simulink model "Actuator_Bench_CAN"  (R2014b)
settings: Solver=ode4  StartTime=0.0  StopTime=Inf  FixedStep=0.001  RelTol=1e-3
PostLoadFcn:
  | , if any(exist('dsrtsu_mdlpostloadfcn', 'file') == [2, 3, 6]), try dsrtsu_mdlpostloadfcn('Execute', bdroot); catch fprintf('Error in PostLoadFcn (dsrtsu_mdlpostloadfcn) for model "%s":\n %s\n', bdroot, lasterr); end, end,
undefined symbols (not defined in the file or in its folder): rticanmm_blockfcn, rticanmm_initfcn
libraries: rtimmsu_dsrtlib x2
settings Model: DSRTSU_INTERNAL_RTI_VER=450  DSRTSU_INTERNAL_RTI_TYPE=rti1401  RTICANMMDATA=struct('GeneralSetupData',struct('modelroot','F:\Clutch','generalsettings',struct('filesettings',struct('destfolder',struct('Name','RTICANMM_FILES','Check',1),'buildfolder',struct('Name','.','Check',1),'AbsDestfolder',struct('Name','F:\Clutch\RTICANMM_FILES'),'AbsBuildfolder',struct('Name','F:\Clutch'))),'options',struct('addpaths',1,'rmpaths',1,'addtrcexclusion',logical(1),'cannavigator',struct('checkmonitoring',0,'checkinternmonitoring',1,'serviceno','31','hostservicedefheader',struct('name','RTICANMMHostService_Lesson1_TutorialModel.h','path','E:\Lessons_Tutorial\Lesson1_results\RTICANMMTutorial\RTICANMM_FILES\RTICANMMHostService_Lesson1_TutorialModel.h')),'show_usrtrc',0,'use_usrtrc',0,'addpath2usrmk',1),'advanced',struct('options',[1 1 1 1 1 1 1 1 1 1 1 1 1 1 1 1 1 1 1 1 1 1 1 1 1 1 1 1 1 1 1 1 1 1 1 1 1 1 1 1 1 1 1 1 1 1 1 1 1 1 1 1 1 1 1 1 1 1 1 1 1 1 1 1 1 1 1 1 1 1 1 1 1 1 1 1 1 1 1 1 1 1 1 1 1 1 1 1 1 1 1 1 1 1 1 1 1 1 1 1]),'MPSetup',{{}},'modelname','Actuator_Bench_CAN2','blockdata',struct('generalsettings',struct('filesettings',struct('destfolder',struct('Name','.','Check',1),'AbsDestfolder',struct('Name','T:\TOOL_SOURCES\CANnedy\m'),'buildfolder',struct('Name','.','Check',1),'AbsBuildfolder',struct('Name','C:\MATLAB6p5\work'))),'options',struct('addpaths',1,'rmpaths',1,'addpath2usrmk',1),'modelname','rticanmmlib','modelroot','T:\TOOL_SOURCES\CANnedy\m'),'userdata',struct('CANMMName',{{'Chassis_M1','Chassis_M2'}},'HostServiceChannelID',{{'ACTUATOR_CAN',[],[],[],[]}}),'RTI',struct('Type','RTI1401','Ver','7.3','Date','02-Nov-2014'),'version','4.0.735878.5444907408','MMType','RTICANMM','block',['Actuator_Bench_CAN2/RTICANMM' char(10) 'GeneralSetup']))  DSRTSU_INTERNAL_RTIFPGA=40  BufferReuse=off  Creator=Burninator  LastModifiedBy=Stealth
settings OptimizationCC: BlockReduction=off  OptimizeBlockIOStorage=off  BufferReuse=off  GlobalBufferReuse=off  ExpressionFolding=off  LocalBlockOutputs=off
settings HardwareCC: ProdIntDivRoundTo=Zero  ProdEndianess=BigEndian  ProdHWDeviceType=Generic->Custom  TargetIntDivRoundTo=Zero  TargetEndianess=BigEndian  TargetHWDeviceType=Generic->Custom
settings RTWCC: SystemTargetFile=rti1401.tlc  MakeCommand=make_rti  TemplateMakefile=rti1401.tmf  Description=dSPACE DS1401 Hardware Platform  ProcessScript=rti1401_make_rtw_hook
settings STFCustomTargetCC: ParMdlRefBuildCompliant=on  GeneratePreprocessorConditionals=Disable all  SystemTargetFile=rti1401.tlc
settings GRTTargetCC: CompOptLevelCompliant=off  ConcurrentExecutionCompliant=off  CombineOutputUpdateFcns=off  MatFileLogging=off  CPPClassGenCompliant=off  GRTInterface=on  ExtModeMexFile=noextcomm

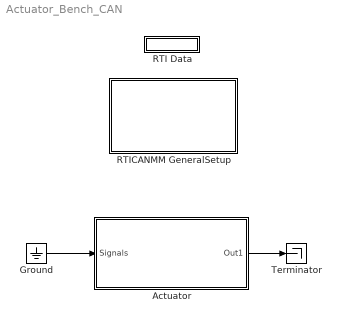
== system Actuator_Bench_CAN ==
  Actuator : Subsystem
  Ground : Ground
  RTI Data : Subsystem  Tag=struct('RTIDataServer',struct('RTIDataServerVs','2','RTIModelDescription','struct(''main'',''Actuator_Bench_CAN2'',''sub'','''',''isMp'',0)'))  LoadFcn="if exist('rtidc'), try,  rtidc('DataHostBlockClbLoad', gcbh); catch, disp(['Warning: ''LoadFcn'' for RTI Data block failed: ' lasterr]); end, end,"  mask(RTI_DATA_HOST){}
      mask help:
      | RTI Data Block.
      | This block is used by RTI to store internal model-dependent data.
      | Please keep this block on the root level of the model. Deleting this block will result in data loss.
      |
      | NEVER DELETE OR COPY THIS BLOCK!
      settings: CopyFcn="if exist('rtidc'), try,  rtidc('DataHostBlockClbCopy', gcbh); catch, disp(['Warning: ''CopyFcn'' for RTI Data block failed: ' lasterr]); end, end,"  DeleteFcn="if exist('rtidc'), try,  rtidc('DataHostBlockClbDelete', gcbh); catch, disp(['Warning: ''DeleteFcn'' for RTI Data block failed: ' lasterr]); end, end,"  ModelCloseFcn="if exist('rtidc'), try,  rtidc('DataHostBlockClbModelClose', gcbh); catch, disp(['Warning: ''ModelCloseFcn'' for RTI Data block failed: ' lasterr]); end, end,"  PreSaveFcn="if exist('rtidc'), try,  rtidc('DataHostBlockClbPreSave', gcbh); catch, disp(['Warning: ''PreSaveFcn'' for RTI Data block failed: ' lasterr]); end, end,"  PostSaveFcn="if exist('rtidc'), try,  rtidc('DataHostBlockClbPostSave', gcbh); catch, disp(['Warning: ''PostSaveFcn'' for RTI Data block failed: ' lasterr]); end, end,"  NameChangeFcn="if exist('rtidc'), try,  rtidc('DataHostBlockClbNameChange', gcbh); catch, disp(['Warning: ''NameChangeFcn'' for RTI Data block failed: ' lasterr]); end, end,"
      mask Help:
      | RTI Data Block.
      | This block is used by RTI to store internal model-dependent data.
      | Please keep this block on the root level of the model. Deleting this block will result in data loss.
      | 
      | NEVER DELETE OR COPY THIS BLOCK!
      mask Display:
      | text(0.5, 0.5, 'RTI Data', 'HorizontalAlignment', 'center');
      | plot([1 0]);
  RTICANMM GeneralSetup : Subsystem  InitFcn=rticanmm_initfcn(gcb, 'CANnedySettings')  ClipboardFcn=rticanmm_blockfcn('ClipboardFcn', 'CANnedySettings', gcb)  mask(RTICANMM){DSProperties=struct('RTI',struct('Version',uint32(1),'BlockType',struct('isSLSource',uint8(1),'isSLSink',uint8(1),'isHWSource',uint8(0),'isHWSink',uint8(0),'isSetup',uint8(0),'isInline',uint8(1),'isNonInline',uint8(0),'isInterrupt',uint8(0),'isChannelwise',uint8(0)),'IOBoardType','RTICANMM','UnitType','RTICANMM','Identifier','GENERALSETUP','DialogType','SL','BlockSet','RTICANMM','SlaveProcessor','CAN')), CANMMDestFolder=RTICANMM_FILES, CANMMBuildDir=., CANMMAddPaths=on, CANMMAddpathUserMake=on, CANMMRemovePathOnclose=on, CANMMType=CANnedySettings, CANMMProperties=struct('modelroot','F:\Clutch','generalsettings',struct('filesettings',struct('destfolder',struct('Name','RTICANMM_FILES','Check',1),'buildfolder',struct('Name','.','Check',1),'AbsDestfolder',struct('Name','F:\Clutch\RTICANMM_FILES'),'AbsBuildfolder',struct('Name','F:\Clutch'))),'options',struct('addpaths',1,'rmpaths',1,'addtrcexclusion',logical(1),'cannavigator',struct('checkmonitoring',0,'checkinternmonitoring',1,'serviceno','31','hostservicedefheader',struct('name','RTICANMMHostService_Lesson1_TutorialModel.h','path','E:\Lessons_Tutorial\Lesson1_results\RTICANMMTutorial\RTICANMM_FILES\RTICANMMHostService_Lesson1_TutorialModel.h')),'show_usrtrc',0,'use_usrtrc',0,'addpath2usrmk',1),'advanced',struct('options',[1 1 1 1 1 1 1 1 1 1 1 1 1 1 1 1 1 1 1 1 1 1 1 1 1 1 1 1 1 1 1 1 1 1 1 1 1 1 1 1 1 1 1 1 1 1 1 1 1 1 1 1 1 1 1 1 1 1 1 1 1 1 1 1 1 1 1 1 1 1 1 1 1 1 1 1 1 1 1 1 1 1 1 1 1 1 1 1 1 1 1 1 1 1 1 1 1 1 1 1]),'MPSetup',{{}},'modelname','Actuator_Bench_CAN2','blockdata',struct('generalsettings',struct('filesettings',struct('destfolder',struct('Name','.','Check',1),'AbsDestfolder',struct('Name','T:\TOOL_SOURCES\CANnedy\m'),'buildfolder',struct('Name','.','Check',1),'AbsBuildfolder',struct('Name','C:\MATLAB6p5\work'))),'options',struct('addpaths',1,'rmpaths',1,'addpath2usrmk',1),'modelname','rticanmmlib','modelroot','T:\TOOL_SOURCES\CANnedy\m'),'userdata',struct('CANMMName',{{'Chassis_M1','Chassis_M2'}},'HostServiceChannelID',{{'ACTUATOR_CAN',[],[],[],[]}}),'RTI',struct('Type','RTI1401','Ver','7.3','Date','02-Nov-2014'),'version','4.0.735878.5444907408','MMType','RTICANMM','block',['Actuator_Bench_CAN2/RTICANMM' char(10) 'GeneralSetup'])}
      mask prompts: CANMMDestFolder "Destination Folder for generated Files:"; CANMMBuildDir "Build Directory (*_usr.mk, *_usr.trc)"; CANMMAddPaths "Add Paths automatically"; CANMMAddpathUserMake "Add Paths to UserMake-File"; CANMMRemovePathOnclose "Remove added Path on ModelClose"
      mask init:
      | rticanmm_initfcn(gcb,'CANnedyGeneralSettings')
      settings: CopyFcn=rticanmm_blockfcn('CopyFcn', 'CANnedySettings', gcb)  DeleteFcn=rticanmm_blockfcn('DeleteFcn', 'CANnedySettings', gcb)  ModelCloseFcn=rticanmm_blockfcn('CloseFcn', 'CANnedyGeneralSettings', gcb)  NameChangeFcn=rticanmm_blockfcn('NameChangeFcn', 'CANnedySettings', gcb)  OpenFcn=try, rticanmm_gs_gui('create',gcb), ; catch,errordlg({lasterr, '','Please check your RTI installation.'},['Error: ' upper(bdroot)], 'replace'); end  MoveFcn=rticanmm_blockfcn('MoveFcn', 'CANnedySettings', gcb)
      mask Help: eval('rticanmm_quickstart(''create'', gcb);', 'disp(lasterr);')
      mask Display: disp(sprintf(['RTI CAN\nMultiMessage\nGeneralSetup']))
  Terminator : Terminator
  wires:
  Actuator/1(Out1) -> Terminator/1
  Ground/1 -> Actuator/1(Signals)

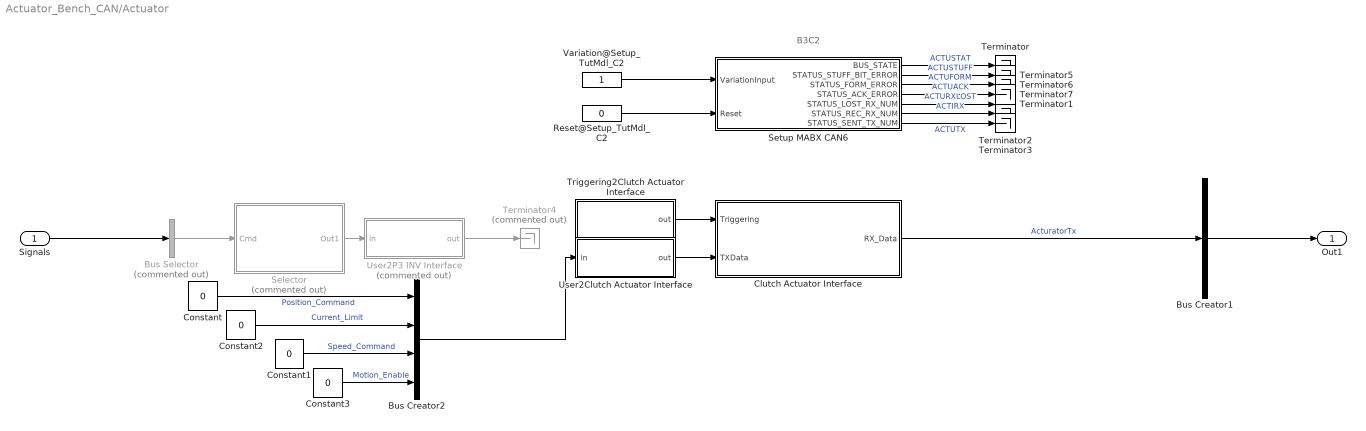
== system Actuator_Bench_CAN/Actuator ==
  note: B3C2
  Signals : Inport
  Bus Creator1 : BusCreator  Inputs=1
  Bus Creator2 : BusCreator
  Bus Selector : BusSelector  Commented=on  OutputSignals=ExecutiveCommands.ComponentStateControl.P3InvCtrl.InverterEnable[Flag],ExecutiveCommands.ComponentStateControl.P3InvCtrl.DischargeEnable[Flag],ExecutiveCommands.ComponentStateControl.P3InvCtrl.Direction[Flag],ExecutiveCommands.TorqueControl.P3Trq.P3TorqueCommand[Nm]  OutputAsBus=on
  Clutch Actuator Interface : Subsystem  InitFcn=rticanmm_blockfcn('InitFcn', 'CANnedy', gcb)  ClipboardFcn=rticanmm_blockfcn('ClipboardFcn', 'CANnedy', gcb)  mask(RTICANMM){DSProperties=struct('RTI',struct('Version',uint32(1),'BlockType',struct('isSLSource',uint8(1),'isSLSink',uint8(1),'isHWSource',uint8(0),'isHWSink',uint8(0),'isSetup',uint8(0),'isInline',uint8(1),'isNonInline',uint8(0),'isInterrupt',uint8(0),'isChannelwise',uint8(0)),'IOBoardType','RTICANMM','UnitType','RTICANMM','Identifier','Mainblock','DialogType','SL','BlockSet','RTICANMM','SlaveProcessor','CAN')), CANMMProperties=struct('RTICANMMVersion','4.0','RTICANMMVersionIntern','4.0.735878.5444907408','RTICANMMDate','02-Nov-2014','Settings','RTICANMM_MAIN_CAN6','UserTracePath','','ModelPath','F:\Clutch','filesettings',struct('FileName','Clutch.dbc','IsRelative',1,'ClusterId',1,'ClusterList',{{'default'}},'destfolder',struct('Name','RTICANMM_FILES','Check',1),'buildfolder',struct('Name','.','Check',1),'onlyfreerawcapture',0,'overlapping2variant',0,'canfdsupport',0),'onlyfreerawcapture',0,'Board',['CAN Type 1'],'BoardNum','3','ChannelNum','2','Variation','1','SetupId','ACTUATOR_CAN','MARK',['4B451E4CC965ABA1126FF18852ACAC';'52181FAC453988346E72CD977C4BB0';'1EB0637A588B713B34B1F65E3CCCD4';'7A7D1E3C4C054BB56A755C5D40C18B';'1806BA38BE006B3F777393E4A2C54E'],'date','06-Jan-2017','clock',['06.01.2017 16:38:25'],'recreate',0,'RTIVER','RTI1401','j1939',0,'TRC',struct('include',1),'rtsupport',struct('XMLFile','F:\Clutch\RTICANMM_FILES\RTICANMM_MAIN_CAN6.xml','DBCXML',struct('Path','F:\Clutch\RTICANMM_FILES\RTICANMM_MAIN_CAN6_dbc.xml','support',1,'Name','Clutch.dbc','Date',['06-Jan-2017 16:32:48'],'Type','extended','DBCSupport','ON'))), CANMMType=CANnedy, CANMMUserTraceMerged=off, CANMMUserTracePath=, CANMMChannelNum=2, CANMMBoardNum=3, CANMMDestFolder=RTICANMM_FILES, CANMMFolder=., CANMMSetupId=ACTUATOR_CAN, CANMMsave2mat=['4B451E4CC965ABA1126FF18852ACAC';'52181FAC453988346E72CD977C4BB0';'1EB0637A588B713B34B1F65E3CCCD4';'7A7D1E3C4C054BB56A755C5D40C18B';'1806BA38BE006B3F777393E4A2C54E'], CANMMName=CAN6, CANMMSettings=RTICANMM_MAIN_CAN6, CANMMIntermediateTag=RTICANMM_MAIN_CAN6_intermediate, CANMMsfcnname=RTICANMM_MAIN_CAN6}
      mask init:
      | rticanmm_initfcn(gcb, CANMMType, CANMMsfcnname)
      settings: AttributesFormatString=ACTUATOR_CAN[CAN6]: DS1401_B3_C2_V1  CopyFcn=rticanmm_blockfcn('CopyFcn', 'CANnedy', gcb)  DeleteFcn=rticanmm_blockfcn('DeleteFcn', 'CANnedy', gcb)  ModelCloseFcn=rticanmm_blockfcn('ModelCloseFcn', 'CANnedy', gcb)  NameChangeFcn=rticanmm_blockfcn('NameChangeFcn', 'CANnedy', gcb)  OpenFcn=try, rticanmm_main_gui('create',gcb); ; catch,errordlg({lasterr, '','Please check your RTI installation.'},['Error: ' upper(bdroot)], 'replace'); end  MoveFcn=rticanmm_blockfcn('MoveFcn', 'CANnedy', gcb)
      mask Help: eval('rticanmm_quickstart(''create'', gcb);', 'disp(lasterr);')
      mask Display:
      | disp(sprintf('RTI CAN\nMultiMessage\nMainSetup'))
      | port_label('input', 1, 'Triggering')
      | port_label('input', 2, 'TX Data')
      | port_label('output', 1, 'RX Data')
  Constant{,1..3} (4 alike) : Constant  Value=0
  Reset@Setup_TutMdl_C2 : Constant  Value=0  OutDataTypeStr=boolean
  Selector : Subsystem  Commented=on
  Setup MABX CAN6 : Subsystem  InitFcn=rticanmm_blockfcn('InitFcn', 'CANnedySetup', gcb)  ClipboardFcn=rticanmm_blockfcn('ClipboardFcn', 'CANnedySetup', gcb)  mask(RTICANMM){DSProperties=struct('RTI',struct('Version',uint32(1),'BlockType',struct('isSLSource',uint8(1),'isSLSink',uint8(1),'isHWSource',uint8(0),'isHWSink',uint8(0),'isSetup',uint8(0),'isInline',uint8(1),'isNonInline',uint8(0),'isInterrupt',uint8(0),'isChannelwise',uint8(0)),'IOBoardType','RTICANMM','UnitType','RTICANMM','Identifier','BUSSETUP','DialogType','SL','BlockSet','RTICANMM','SlaveProcessor','CAN')), CANMMProperties=struct('cannedy',struct('data',struct('options',struct('controllername','ACTUATOR_CAN','controllernameautomatic',[],'loglevel','0','checkrealtime',0,'checkchangebaudrate',0,'sampletime','1.000','CANControllerStatus',1,'NumberofStuffErr',1,'NumberofFormErr',1,'NumberofAckErr',1,'NumberofBit0Err',0,'NumberofsuccrecRX',1,'Numberofsuccsent',1,'NumberofBit1Err',0,'NumberofCRCErr',0,'NumberoflostRX',1,'Busoff',0,'Busload',0,'OperationPending',0,'TxRetryCount',3,'addtrcexclusion',logical(1),'cannavigator',struct('checkmonitoring',0,'checkinternmonitoring',0),'show_usrtrc',0,'use_usrtrc',0,'checkchangebaudrateFD',0),'modelroot','E:\Lessons_Tutorial\Lesson10_results\RTICANMMTutorial','generalsettings',struct('setupdata',struct('board',['CAN Type 1'],'boardno',3,'channelno',2,'Type','EXT','transceiver','ISO11898-2','busconfig','0x0','feedthrough','false','resistance',struct('r120',1,'roff',0,'r16',1,'r10',0),'baudrate','250','Frequency',[24 36],'samplemode',1,'commChannelTJA1041',6,'config',struct('standard',1,'advanced',0,'register',struct('btr0','0xC1','btr1','0x6F','sp','70','sjw','3','tseg1','15','tseg2','6','brp','1','smpl','0','btr0_36','0xC2','btr1_36','0x6F','sp_36','70','sjw_36','3','tseg1_36','15','tseg2_36','6','brp_36','2','smpl_36','0','btr0_64','0x47','btr1_64','0x1C','sp_64','87','sjw_64','1','tseg1_64','12','tseg2_64','1','brp_64','7','smpl_64','0')),'channelcfg',struct('INTENDISABLE','CAN_INT_DISABLE','intenable',0),'SETUPID','RTICANMM_ACTUATOR_CAN_ID','CONTROLLER_ID','CANMM_CTL_SETUP_ACTUATOR_CAN','mainblock_includefile','RTICANMM_SETUP_ACTUATOR_CAN','canfdenable',0,'canfdboardselected',0,'slotno',1,'moduletype','DS4342','baudrateFD','4000','termination','TERMINATION_ON'),'filesettings',struct('destfolder',struct('Name','RTICANMM_FILES','Check',1),'buildfolder',struct('Name','.','Check',1))),'advanced',struct('options',[1 1 1 1 1 1 1 1 1 1 1 1 1 1 1 1 1 1 1 1 1 1 1 1 1 1 1 1 1 1 1 1 1 1 1 1 1 1 1 1 1 1 1 1 1 1 1 1 1 1 1 1 1 1 1 1 1 1 1 1 1 1 1 1 1 1 1 1 1 1 1 1 1 1 1 1 1 1 1 1 1 1 1 1 1 1 1 1 1 1 1 1 1 1 1 1 1 1 1 1]),'partialnetdata',struct('switchedon',0,'format','STD','idmask',['XXXXX XXXXXXXX XXXXXXXX XXXXXXXX'],'idcode','0','idfilter','0','datamaskused',0,'datalength','0','datamask','0x0000000000000000','partialnetworkenable',0)),'blk',['Actuator_Bench_CAN2/Actuator/Setup MABX CAN6'],'allgeneratedfiles',{{'F:\Clutch\RTICANMM_FILES\RTICANMM_SETUP_ACTUATOR_CAN.c','F:\Clutch\RTICANMM_FILES\RTICANMM_SETUP_ACTUATOR_CAN.h','f:\clutch\rticanmm_files\rticanmm_setup_actuator_can.mexw64'}},'ismp',logical(0),'BlockDataVersion','0.7.0','recreate',0,'CANnedyTag','ACTUATOR_CAN'),'CANnedynew',0,'CANnedySettings','ACTUATOR_CAN','GeneratedFiles',{{'F:\Clutch\RTICANMM_FILES\RTICANMM_SETUP_ACTUATOR_CAN.c','F:\Clutch\RTICANMM_FILES\RTICANMM_SETUP_ACTUATOR_CAN.h','f:\clutch\rticanmm_files\rticanmm_setup_actuator_can.mexw64'}},'SFCN','RTICANMM_SETUP_ACTUATOR_CAN.c','HostService',struct('Tags',struct('DATA','RTICANMM_MonitorData','TimeStampGlobal','RTICANMM_MonitoringTimeStamp','TimeStampGlobalEnable','RTICANMM_MonitoringTimeStampEnable','Enable','CANMMMonitor_ACTUATOR_CAN','TimeStamp','MonitoringTimeStamp_ACTUATOR_CAN'),'DATA',struct('Length',18),'Info',struct('Desc',{'ID','Service','Data1','Data2','Data3','Data4','Data5','Data6','Data7','Data8','Data9','Data10','Data11','Data12','Data13','Data14','Data15','Data16'}),'Names',struct('TimeStampGlobal','TimeStamp','TimeStampGlobalEnable','TimeStamp_Enable','Enable','Monitoring_Enable','TimeStamp','Monitoring_TimeStamp'),'ChannelID',1)), CANMMType=CANnedySetup, CANMMFolder=F:\Clutch, CANMMDestFolder=RTICANMM_FILES, CANMMSettings=ACTUATOR_CAN, CANMMSFcn=RTICANMM_SETUP_ACTUATOR_CAN, CANMMBoard=DS1401, CANMMBoardNum=3, CANMMChannel=2}
      settings: AttributesFormatString=%<CANMMSettings>: %<CANMMBoard>_B%<CANMMBoardNum>_C%<CANMMChannel>  CopyFcn=rticanmm_blockfcn('CopyFcn', 'CANnedySetup', gcb)  DeleteFcn=rticanmm_blockfcn('DeleteFcn', 'CANnedySetup', gcb)  ModelCloseFcn=rticanmm_blockfcn('ModelCloseFcn', 'CANnedySetup', gcb)  NameChangeFcn=rticanmm_blockfcn('NameChangeFcn', 'CANnedySetup', gcb)  OpenFcn=try, rticanmm_setup_gui('create',gcb); ; catch,errordlg({lasterr, '','Please check your RTI installation.'},['Error: ' upper(bdroot)], 'replace'); end  MoveFcn=rticanmm_blockfcn('MoveFcn', 'CANnedySetup', gcb)
      mask Help: eval('rticanmm_quickstart(''create'', gcb);', 'disp(lasterr);')
      mask Display:
      | disp('RTI CAN\nMultiMessage\nControllerSetup')
      | 
      | port_label('input', 1 , 'Variation')
      | port_label('input', 2 , 'Reset')
      | port_label('output', 1, 'Status')
      | port_label('output', 2, 'Stuff errors')
      | port_label('output', 3, 'Format errors')
      | port_label('output', 4, 'Ack errors')
      | port_label('output', 5, 'RX lost')
      | port_label('output', 6, 'RX ok')
      | port_label('output', 7, 'TX ok')
  Terminator{,1..3,5..7} (7 alike) : Terminator
  Terminator4 : Terminator  Commented=on
  Triggering2Clutch Actuator Interface : Subsystem
      mask Display: disp('Triggering\nto RTICANMM')
  User2Clutch Actuator Interface : Subsystem
      mask Display: disp('Mapping\nto RTICANMM')
  User2P3 INV Interface : Subsystem  Commented=on
      mask Display: disp('Mapping\nto RTICANMM')
  Variation@Setup_TutMdl_C2 : Constant  OutDataTypeStr=uint8
  Out1 : Outport
  wires:
  Bus Selector/1 -> Selector/1(Cmd)
  User2P3 INV Interface/1(out) -> Terminator4/1
  Clutch Actuator Interface/1(RX_Data) -> Bus Creator1/1  "ActuratorTx"
  Signals/1 -> Bus Selector/1
  Variation@Setup_TutMdl_C2/1 -> Setup MABX CAN6/1(VariationInput)
  Reset@Setup_TutMdl_C2/1 -> Setup MABX CAN6/2(Reset)
  Bus Creator1/1 -> Out1/1
  Selector/1(Out1) -> User2P3 INV Interface/1(in)
  Setup MABX CAN6/1(BUS_STATE) -> Terminator/1  "ACTUSTAT"
  Setup MABX CAN6/5(STATUS_LOST_RX_NUM) -> Terminator1/1  "ACTURXLOST"
  Setup MABX CAN6/6(STATUS_REC_RX_NUM) -> Terminator2/1  "ACTIRX"
  Setup MABX CAN6/7(STATUS_SENT_TX_NUM) -> Terminator3/1  "ACTUTX"
  Setup MABX CAN6/4(STATUS_ACK_ERROR) -> Terminator7/1  "ACTUACK"
  Setup MABX CAN6/3(STATUS_FORM_ERROR) -> Terminator6/1  "ACTUFORM"
  Setup MABX CAN6/2(STATUS_STUFF_BIT_ERROR) -> Terminator5/1  "ACTUSTUFF"
  Constant/1 -> Bus Creator2/1  "Position_Command"
  Bus Creator2/1 -> User2Clutch Actuator Interface/1(in)
  Constant2/1 -> Bus Creator2/2  "Current_Limit"
  Constant1/1 -> Bus Creator2/3  "Speed_Command"
  Constant3/1 -> Bus Creator2/4  "Motion_Enable"
  Triggering2Clutch Actuator Interface/1(out) -> Clutch Actuator Interface/1(Triggering)
  User2Clutch Actuator Interface/1(out) -> Clutch Actuator Interface/2(TXData)

== system Actuator_Bench_CAN/RTI Data ==
  RTI Data Store : Subsystem  Tag="struct('private',struct('version',struct('dsVer',uint32(2),'dsVerCreation',uint32(2),'RTI',struct('ver','7.3','type','RTI1401')),'access',struct('type','Model','isPerm',1,'created',['06-Jan-2017 09:05:07'],'modified',['06-Jan-2017 16:41:17'],'location','')),'public',struct('main',struct('data',[]),'sub',struct('name',{{'Actuator_Bench_CAN2'}},'data',{{struct('TH',struct('thTaskInfo',struct('taskType',{'TIMER','HWINT','TMRINT','SWINT','GLINT'},'tasksNumOf',{1,0,0,0,0},'srcIds',{{'TIMERA'},{},{},{},{}},'taskNames',{{['Timer Task 1']},{},{},{},{}})),'th_tc',struct('dataType','TASK','taskGroupId','','taskGroupList',{{}},'taskSchedulingPolicy','FCFS','taskType','TIMER','blkh',-1,'srcId','TIMERA','srcSgnName',['Timer A interrupt'],'srcCpuName','','taskName',['Timer Task 1  [0.001] s'],'taskNameDisplayExt','','smplTime',0.001,'smplTimeOffs',0,'hasFixedPriority',0,'priority',1,'hasFixedOvc',0,'ovcType',1,'ovcMax',1),'tc_th',struct('dataType','TASK','taskGroupId','','taskGroupList',{{}},'taskSchedulingPolicy','FCFS','taskType','TIMER','blkh',-1,'srcId','TIMERA','srcSgnName',['Timer A interrupt'],'srcCpuName','','taskName',['Timer Task 1  [0.001] s'],'taskNameDisplayExt','','smplTime',0.001,'smplTimeOffs',0,'hasFixedPriority',0,'priority',1,'hasFixedOvc',0,'ovcType',1,'ovcMax',1))}})))"  mask(RTI_DATA_STORE){}
      mask help:
      | RTI Data Store Block. This block is used by RTI to store internal model dependent data. Deleting this block will result in data loss.
      |
      | NEVER DELETE, COPY, OR MODIFY THIS BLOCK!
      mask Help:
      | RTI Data Store Block. This block is used by RTI to store internal model dependent data. Deleting this block will result in data loss.
      | 
      | NEVER DELETE, COPY, OR MODIFY THIS BLOCK!
      mask Display: text(0.5, 0.5, ' ', 'HorizontalAlignment', 'center');

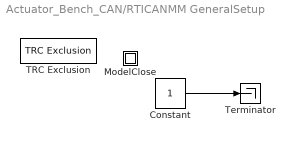
== system Actuator_Bench_CAN/RTICANMM GeneralSetup ==
  Constant : Constant
  ModelClose : Subsystem  mask(RTICANMMModelClose){}
  TRC Exclusion : rtimmsu_dsrtlib/TRC Exclusion
  Terminator : Terminator
  wires:
  Constant/1 -> Terminator/1

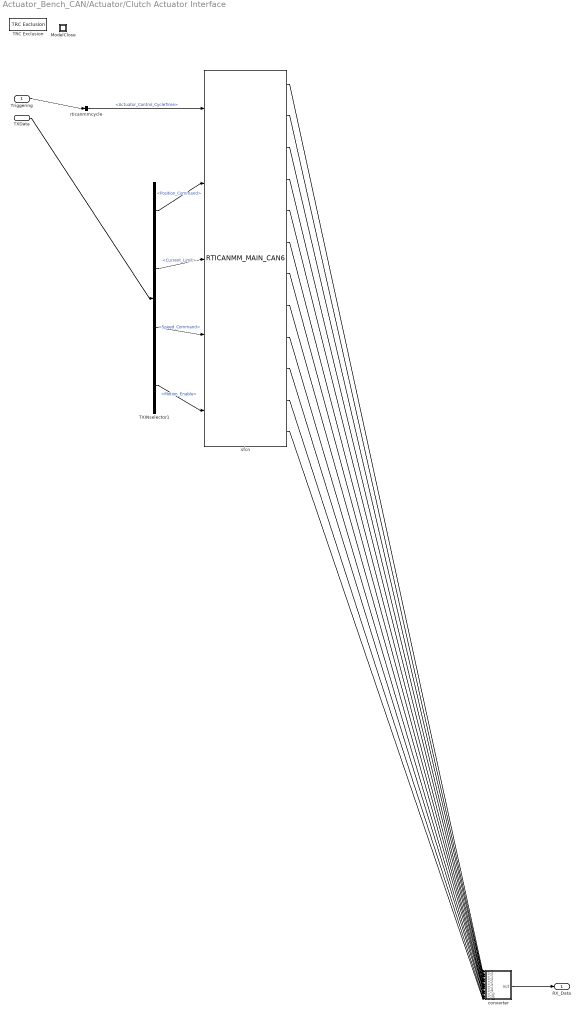
== system Actuator_Bench_CAN/Actuator/Clutch Actuator Interface ==
  Triggering : Inport
  TXData : Inport  Port=2
  ModelClose : Subsystem  mask(RTICANMMModelClose){}
  TRC Exclusion : rtimmsu_dsrtlib/TRC Exclusion
  TXINselector1 : BusSelector  OutputSignals=Actuator_Control.Position_Command,Actuator_Control.Current_Limit,Actuator_Control.Speed_Command,Actuator_Control.Motion_Enable
  converter : Subsystem  mask(CANnedyVector2Bus){}
      mask help: Do not change.
      mask Display: disp('Vector to\nBus')
  rticanmmcycle : BusSelector  OutputSignals=Actuator_Control.Actuator_Control_CycleTime
  sfcn : S-Function  InitFcn=rticanmm_initfcn(gcb, 'SFCNs')  FunctionName=RTICANMM_MAIN_CAN6  EnableBusSupport=off
      mask init:
      | rticanmm_initfcn(gcb, 'SFCNs')
  RX_Data : Outport
  wires:
  Triggering/1 -> rticanmmcycle/1
  rticanmmcycle/1 -> sfcn/1  "<Actuator_Control_CycleTime>"
  TXData/1 -> TXINselector1/1
  TXINselector1/1 -> sfcn/2  "<Position_Command>"
  TXINselector1/2 -> sfcn/3  "<Current_Limit>"
  TXINselector1/3 -> sfcn/4  "<Speed_Command>"
  TXINselector1/4 -> sfcn/5  "<Motion_Enable>"
  converter/1(out) -> RX_Data/1
  sfcn/1 -> converter/1(in_1)
  sfcn/2 -> converter/2(in_2)
  sfcn/3 -> converter/3(in_3)
  sfcn/4 -> converter/4(in_4)
  sfcn/5 -> converter/5(in_5)
  sfcn/6 -> converter/6(in_6)
  sfcn/7 -> converter/7(in_7)
  sfcn/8 -> converter/8(in_8)
  sfcn/9 -> converter/9(in_9)
  sfcn/10 -> converter/10(in_10)
  sfcn/11 -> converter/11(in_11)
  sfcn/12 -> converter/12(in_12)

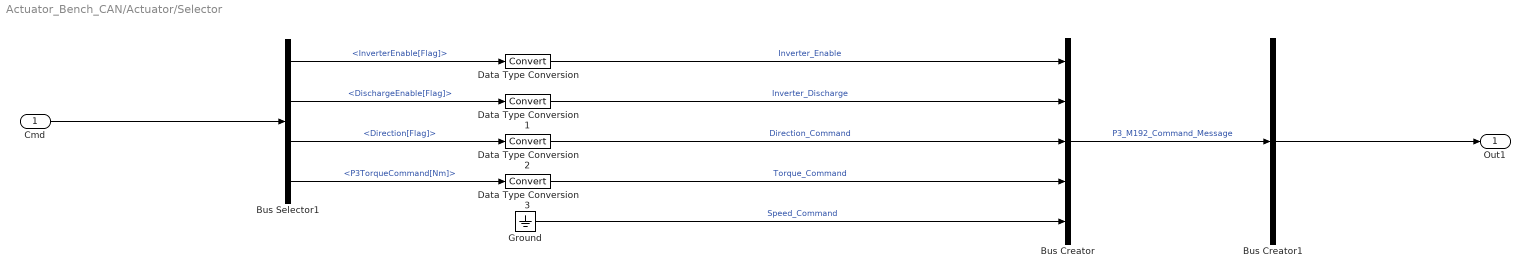
== system Actuator_Bench_CAN/Actuator/Selector ==
  Cmd : Inport
  Bus Creator : BusCreator  Inputs=5
  Bus Creator1 : BusCreator  Inputs=1
  Bus Selector1 : BusSelector  OutputSignals=InverterEnable[Flag],DischargeEnable[Flag],Direction[Flag],P3TorqueCommand[Nm]
  Data Type Conversion{,1..3} (4 alike) : DataTypeConversion
  Ground : Ground
  Out1 : Outport
  wires:
  Cmd/1 -> Bus Selector1/1
  Bus Selector1/1 -> Data Type Conversion/1  "<InverterEnable[Flag]>"
  Bus Selector1/2 -> Data Type Conversion1/1  "<DischargeEnable[Flag]>"
  Bus Selector1/3 -> Data Type Conversion2/1  "<Direction[Flag]>"
  Bus Creator/1 -> Bus Creator1/1  "P3_M192_Command_Message"
  Data Type Conversion1/1 -> Bus Creator/2  "Inverter_Discharge"
  Data Type Conversion2/1 -> Bus Creator/3  "Direction_Command"
  Ground/1 -> Bus Creator/5  "Speed_Command"
  Data Type Conversion3/1 -> Bus Creator/4  "Torque_Command"
  Data Type Conversion/1 -> Bus Creator/1  "Inverter_Enable"
  Bus Creator1/1 -> Out1/1
  Bus Selector1/4 -> Data Type Conversion3/1  "<P3TorqueCommand[Nm]>"

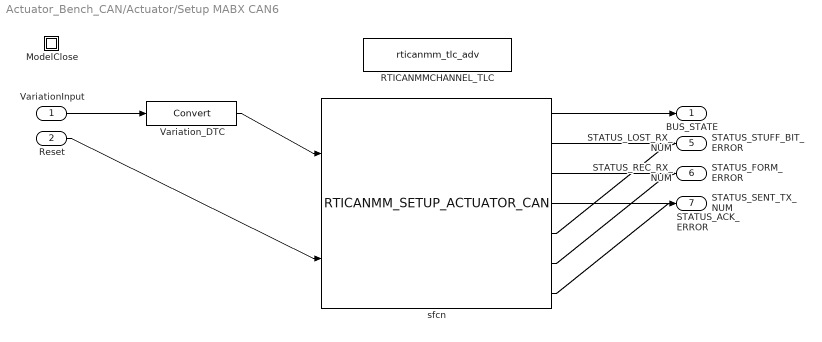
== system Actuator_Bench_CAN/Actuator/Setup MABX CAN6 ==
  VariationInput : Inport
  Reset : Inport  Port=2
  ModelClose : Subsystem  mask(RTICANMMModelClose){}
  RTICANMMCHANNEL_TLC : S-Function  FunctionName=rticanmm_tlc_adv  Parameters=1401,3,2,0,250,'unused'  EnableBusSupport=off  mask(RTICANMMCHANNEL_TLC){}
  Variation_DTC : DataTypeConversion  SaturateOnIntegerOverflow=on  RndMeth=Zero
  sfcn : S-Function  InitFcn=rticanmm_initfcn(gcb, 'SFCNs')  FunctionName=RTICANMM_SETUP_ACTUATOR_CAN  EnableBusSupport=off
      mask init:
      | rticanmm_initfcn(gcb, 'SFCNs')
  BUS_STATE : Outport
  STATUS_STUFF_BIT_ERROR : Outport  Port=2
  STATUS_FORM_ERROR : Outport  Port=3
  STATUS_ACK_ERROR : Outport  Port=4
  STATUS_LOST_RX_NUM : Outport  Port=5
  STATUS_REC_RX_NUM : Outport  Port=6
  STATUS_SENT_TX_NUM : Outport  Port=7
  wires:
  Reset/1 -> sfcn/2
  sfcn/1 -> BUS_STATE/1
  sfcn/2 -> STATUS_STUFF_BIT_ERROR/1
  sfcn/3 -> STATUS_FORM_ERROR/1
  sfcn/4 -> STATUS_ACK_ERROR/1
  sfcn/5 -> STATUS_LOST_RX_NUM/1
  sfcn/6 -> STATUS_REC_RX_NUM/1
  sfcn/7 -> STATUS_SENT_TX_NUM/1
  VariationInput/1 -> Variation_DTC/1
  Variation_DTC/1 -> sfcn/1

== system Actuator_Bench_CAN/Actuator/Triggering2Clutch Actuator Interface ==
  Actuator_Control : Subsystem
  buscreator : BusCreator  Inputs=1
  out : Outport
  wires:
  Actuator_Control/1(out) -> buscreator/1  "Actuator_Control"
  buscreator/1 -> out/1  "CAN"

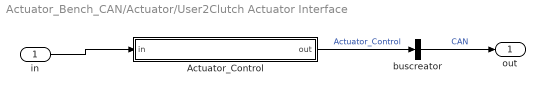
== system Actuator_Bench_CAN/Actuator/User2Clutch Actuator Interface ==
  in : Inport
  Actuator_Control : Subsystem
  buscreator : BusCreator  Inputs=1
  out : Outport
  wires:
  Actuator_Control/1(out) -> buscreator/1  "Actuator_Control"
  in/1 -> Actuator_Control/1(in)
  buscreator/1 -> out/1  "CAN"

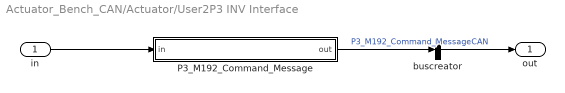
== system Actuator_Bench_CAN/Actuator/User2P3 INV Interface ==
  in : Inport
  P3_M192_Command_Message : Subsystem
  buscreator : BusCreator  Inputs=1
  out : Outport
  wires:
  P3_M192_Command_Message/1(out) -> buscreator/1  "P3_M192_Command_Message"
  in/1 -> P3_M192_Command_Message/1(in)
  buscreator/1 -> out/1  "CAN"

== system Actuator_Bench_CAN/RTI Data/RTI Data Store ==
  RTI Data Store : Subsystem  mask(RTI_DATA_STORE){}
      mask help:
      | RTI Data Store Block. This block is used by RTI to store internal model dependent data. Deleting this block will result in data loss.
      |
      | NEVER DELETE, COPY, OR MODIFY THIS BLOCK!
      mask Help:
      | RTI Data Store Block. This block is used by RTI to store internal model dependent data. Deleting this block will result in data loss.
      | 
      | NEVER DELETE, COPY, OR MODIFY THIS BLOCK!
      mask Display: text(0.5, 0.5, ' ', 'HorizontalAlignment', 'center');

== system Actuator_Bench_CAN/RTICANMM GeneralSetup/ModelClose ==

== system Actuator_Bench_CAN/Actuator/Clutch Actuator Interface/ModelClose ==

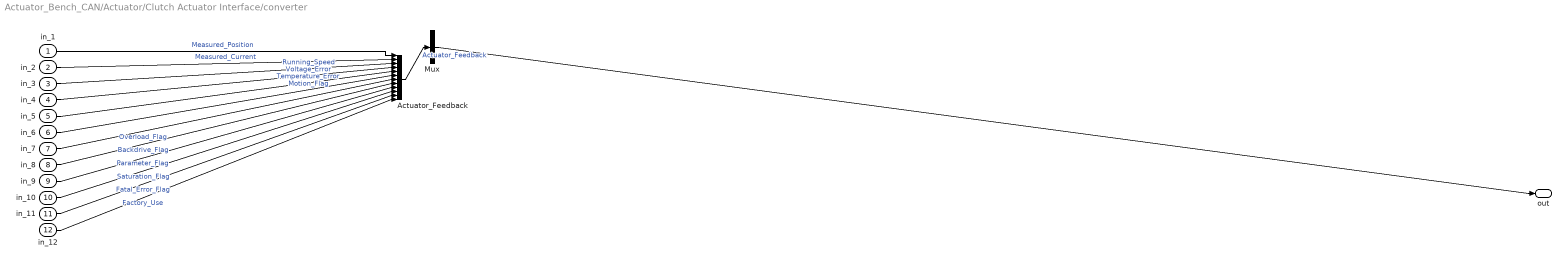
== system Actuator_Bench_CAN/Actuator/Clutch Actuator Interface/converter ==
  in_1 : Inport
  in_2 : Inport  Port=2
  in_3 : Inport  Port=3
  in_4 : Inport  Port=4
  in_5 : Inport  Port=5
  in_6 : Inport  Port=6
  in_7 : Inport  Port=7
  in_8 : Inport  Port=8
  in_9 : Inport  Port=9
  in_10 : Inport  Port=10
  in_11 : Inport  Port=11
  in_12 : Inport  Port=12
  Actuator_Feedback : BusCreator  Inputs=12
  Mux : BusCreator  Inputs=1
  out : Outport
  wires:
  in_1/1 -> Actuator_Feedback/1  "Measured_Position"
  Actuator_Feedback/1 -> Mux/1  "Actuator_Feedback"
  in_2/1 -> Actuator_Feedback/2  "Measured_Current"
  in_3/1 -> Actuator_Feedback/3  "Running_Speed"
  in_4/1 -> Actuator_Feedback/4  "Voltage_Error"
  in_5/1 -> Actuator_Feedback/5  "Temperature_Error"
  in_6/1 -> Actuator_Feedback/6  "Motion_Flag"
  in_7/1 -> Actuator_Feedback/7  "Overload_Flag"
  in_8/1 -> Actuator_Feedback/8  "Backdrive_Flag"
  in_9/1 -> Actuator_Feedback/9  "Parameter_Flag"
  in_10/1 -> Actuator_Feedback/10  "Saturation_Flag"
  in_11/1 -> Actuator_Feedback/11  "Fatal_Error_Flag"
  in_12/1 -> Actuator_Feedback/12  "Factory_Use"
  Mux/1 -> out/1

== system Actuator_Bench_CAN/Actuator/Setup MABX CAN6/ModelClose ==

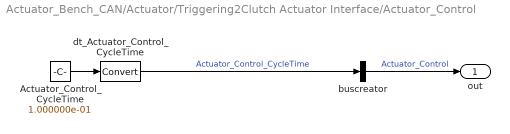
== system Actuator_Bench_CAN/Actuator/Triggering2Clutch Actuator Interface/Actuator_Control ==
  Actuator_Control_CycleTime : Constant  Value=1.000000e-01
  buscreator : BusCreator  Inputs=1
  dt_Actuator_Control_CycleTime : DataTypeConversion  RndMeth=Zero
  out : Outport
  wires:
  buscreator/1 -> out/1  "Actuator_Control"
  Actuator_Control_CycleTime/1 -> dt_Actuator_Control_CycleTime/1
  dt_Actuator_Control_CycleTime/1 -> buscreator/1  "Actuator_Control_CycleTime"

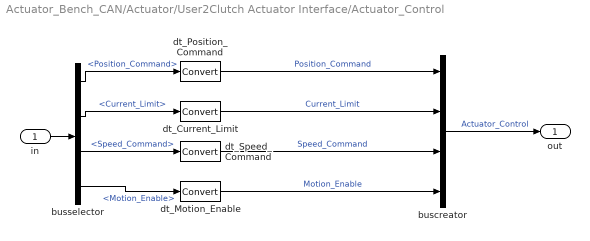
== system Actuator_Bench_CAN/Actuator/User2Clutch Actuator Interface/Actuator_Control ==
  in : Inport
  buscreator : BusCreator
  busselector : BusSelector  OutputSignals=Position_Command,Current_Limit,Speed_Command,Motion_Enable
  dt_Current_Limit : DataTypeConversion  RndMeth=Zero
  dt_Motion_Enable : DataTypeConversion  RndMeth=Zero
  dt_Position_Command : DataTypeConversion  RndMeth=Zero
  dt_Speed_Command : DataTypeConversion  RndMeth=Zero
  out : Outport
  wires:
  buscreator/1 -> out/1  "Actuator_Control"
  in/1 -> busselector/1
  busselector/1 -> dt_Position_Command/1  "<Position_Command>"
  dt_Position_Command/1 -> buscreator/1  "Position_Command"
  busselector/2 -> dt_Current_Limit/1  "<Current_Limit>"
  dt_Current_Limit/1 -> buscreator/2  "Current_Limit"
  busselector/3 -> dt_Speed_Command/1  "<Speed_Command>"
  dt_Speed_Command/1 -> buscreator/3  "Speed_Command"
  busselector/4 -> dt_Motion_Enable/1  "<Motion_Enable>"
  dt_Motion_Enable/1 -> buscreator/4  "Motion_Enable"

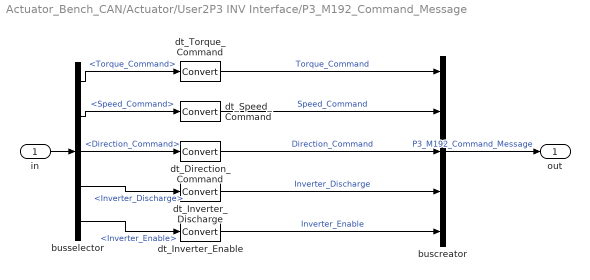
== system Actuator_Bench_CAN/Actuator/User2P3 INV Interface/P3_M192_Command_Message ==
  in : Inport
  buscreator : BusCreator  Inputs=5
  busselector : BusSelector  OutputSignals=P3_M192_Command_Message.Torque_Command,P3_M192_Command_Message.Speed_Command,P3_M192_Command_Message.Direction_Command,P3_M192_Command_Message.Inverter_Discharge,P3_M192_Command_Message.Inverter_Enable
  dt_Direction_Command : DataTypeConversion  RndMeth=Zero
  dt_Inverter_Discharge : DataTypeConversion  RndMeth=Zero
  dt_Inverter_Enable : DataTypeConversion  RndMeth=Zero
  dt_Speed_Command : DataTypeConversion  RndMeth=Zero
  dt_Torque_Command : DataTypeConversion  RndMeth=Zero
  out : Outport
  wires:
  buscreator/1 -> out/1  "P3_M192_Command_Message"
  in/1 -> busselector/1
  busselector/1 -> dt_Torque_Command/1  "<Torque_Command>"
  dt_Torque_Command/1 -> buscreator/1  "Torque_Command"
  busselector/2 -> dt_Speed_Command/1  "<Speed_Command>"
  dt_Speed_Command/1 -> buscreator/2  "Speed_Command"
  busselector/3 -> dt_Direction_Command/1  "<Direction_Command>"
  dt_Direction_Command/1 -> buscreator/3  "Direction_Command"
  busselector/4 -> dt_Inverter_Discharge/1  "<Inverter_Discharge>"
  dt_Inverter_Discharge/1 -> buscreator/4  "Inverter_Discharge"
  busselector/5 -> dt_Inverter_Enable/1  "<Inverter_Enable>"
  dt_Inverter_Enable/1 -> buscreator/5  "Inverter_Enable"

== system Actuator_Bench_CAN/RTI Data/RTI Data Store/RTI Data Store ==
  RTI Data Store : Subsystem  mask(RTI_DATA_STORE){}
      mask help:
      | RTI Data Store Block. This block is used by RTI to store internal model dependent data. Deleting this block will result in data loss.
      |
      | NEVER DELETE, COPY, OR MODIFY THIS BLOCK!
      mask Help:
      | RTI Data Store Block. This block is used by RTI to store internal model dependent data. Deleting this block will result in data loss.
      | 
      | NEVER DELETE, COPY, OR MODIFY THIS BLOCK!
      mask Display: text(0.5, 0.5, ' ', 'HorizontalAlignment', 'center');

== system Actuator_Bench_CAN/RTI Data/RTI Data Store/RTI Data Store/RTI Data Store ==
  RTI Data Store : Subsystem  mask(RTI_DATA_STORE){}
      mask help:
      | RTI Data Store Block. This block is used by RTI to store internal model dependent data. Deleting this block will result in data loss.
      |
      | NEVER DELETE, COPY, OR MODIFY THIS BLOCK!
      mask Help:
      | RTI Data Store Block. This block is used by RTI to store internal model dependent data. Deleting this block will result in data loss.
      | 
      | NEVER DELETE, COPY, OR MODIFY THIS BLOCK!
      mask Display: text(0.5, 0.5, ' ', 'HorizontalAlignment', 'center');

== system Actuator_Bench_CAN/RTI Data/RTI Data Store/RTI Data Store/RTI Data Store/RTI Data Store ==
